simulink model "SimpleMPC"  (R2021a)
settings: Solver=FixedStepAuto  StartTime=0.0  StopTime=T  FixedStep=Ts  RelTol=1e-3
undefined symbols (not defined in the file): A, B, F, N, Q, R, Ts, x0
settings Model: Creator=xiaocy  LastModifiedBy=xiaocy
settings DataIOCC: ReturnWorkspaceOutputs=off

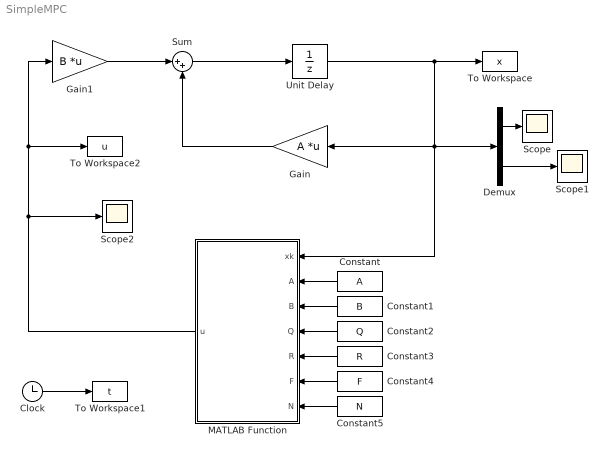
== system SimpleMPC ==
  Clock : Clock
  Constant : Constant  Value=A
  Constant1 : Constant  Value=B
  Constant2 : Constant  Value=Q
  Constant3 : Constant  Value=R
  Constant4 : Constant  Value=F
  Constant5 : Constant  Value=N
  Demux : Demux  Outputs=2
  Gain : Gain  Gain=A  Multiplication=Matrix(K*u)
  Gain1 : Gain  Gain=B  Multiplication=Matrix(K*u)
  MATLAB Function : MATLAB Function  TreatAsAtomicUnit=on  SystemSampleTime=Ts
  Scope : Scope
  Scope1 : Scope
  Scope2 : Scope
  Sum : Sum  Inputs=|++
  To Workspace : ToWorkspace  VariableName=x  SampleTime=-1
  To Workspace1 : ToWorkspace  VariableName=t  SampleTime=-1
  To Workspace2 : ToWorkspace  VariableName=u  SampleTime=-1
  Unit Delay : UnitDelay  InitialCondition=x0  SampleTime=Ts  HasFrameUpgradeWarning=on
  wires:
  Sum/1 -> Unit Delay/1
  Unit Delay/1 -> MATLAB Function/1(xk), Demux/1, Gain/1, To Workspace/1
  Gain1/1 -> Sum/1
  Gain/1 -> Sum/2
  Constant/1 -> MATLAB Function/2(A)
  Constant1/1 -> MATLAB Function/3(B)
  Constant2/1 -> MATLAB Function/4(Q)
  Constant3/1 -> MATLAB Function/5(R)
  Constant4/1 -> MATLAB Function/6(F)
  Constant5/1 -> MATLAB Function/7(N)
  Demux/1 -> Scope/1
  Demux/2 -> Scope1/1
  MATLAB Function/1(u) -> Scope2/1, Gain1/1, To Workspace2/1
  Clock/1 -> To Workspace1/1

== matlab function SimpleMPC/MATLAB Function ==
  data: xk input; u output; A input; B input; Q input; R input; F input; N input
function u = getCmdMPC(xk,A,B,Q,R,F,N)
    n = size(A,1);
    M = eye(n*(N+1),n);
    C = zeros(n*(N+1),N*size(B,2));
    
    Mi = eye(n);
    Bi = B;
    for i = 1:N
        Mi = A*Mi;
        rowM = (i*n+1):(i*n+n);
        M(rowM,:) = Mi;

        if i >= 2
            Bi = A*Bi;
        end

        rowC = (i*n+1):n*(N+1);
        colC = 1:(N+1-i)*size(B,2);
        C(rowC,colC) = C(rowC,colC) + kron(eye(N+1-i),Bi);
    end

    Qbar = blkdiag(kron(eye(N),Q),F);
    Rbar = kron(eye(N),R);
    H = C'*Qbar*C + Rbar;
    f = C'*Qbar'*M*xk;

    % special settings for Simulink
    opts = optimoptions('quadprog','Display','off','Algorithm','active-set');
    U = quadprog(H,f,[],[],[],[],[],[],zeros(size(H,1),1),opts);
    u = U(1);
end
